simulink model "R7014E_DoubleTankSim"  (R2024b)
settings: Solver=ode5  StartTime=0.0  StopTime=2000  FixedStep=Ts  RelTol=1e-3  EnableMultiTasking=on
undefined symbols (not defined in the file): Ad, Bd, Cd, h_10, h_20, K, Q, T, Ts, u0
libraries: simulink x3, cstblocks x1
Description:
  | Double tank process simulation model
  | V1.0
  | 
  | Author: Wolfgang Birk, LTU
settings Model: MinMaxOverflowLogging=ForceOff  Creator=wolfgang  LastModifiedBy=Amar
settings SolverCC: AlgebraicLoopSolver=TrustRegion
settings DataIOCC: LimitDataPoints=on  SaveFormat=Array  SignalLoggingSaveFormat=ModelDataLogs  ReturnWorkspaceOutputs=off
settings OptimizationCC: ExpressionDepthLimit=2147483647  LifeSpan=inf
settings DebuggingCC: UnderspecifiedInitializationDetection=Classic  MergeDetectMultiDrivingBlocksExec=none  SolverPrmCheckMsg=warning  FcnCallInpInsideContextMsg=warning  UnconnectedInputMsg=warning  UnconnectedOutputMsg=warning  UnconnectedLineMsg=warning  StateNameClashWarn=warning  SFUnexpectedBacktrackingDiag=warning  SFNoUnconditionalDefaultTransitionDiag=warning  SFExecutionAtInitializationDiag=none  ArithmeticOperatorsInVariantConditions=warning
settings HardwareCC: ProdBitPerPointer=32  ProdBitPerSizeT=32  ProdBitPerPtrDiffT=32  ProdLargestAtomicFloat=None  ProdIntDivRoundTo=Undefined  ProdEndianess=Unspecified  ProdWordSize=32  ProdHWDeviceType=32-bit Generic
settings ModelReferenceCC: EnableRefExpFcnMdlSchedulingChecks=on  PropagateSignalLabelsOutOfModel=off
settings SFSimCC: SimUseLocalCustomCode=off  CustomCodeUndefinedFunction=UseInterfaceOnly
settings RTWCC: RTWUseLocalCustomCode=off  GPUComputeCapability=3.5
settings CodeAppCC: StateflowObjectComments=on
settings GRTTargetCC: TargetLangStandard=C89/C90 (ANSI)
settings ConfigComp: CovMetricSettings=dw  CovSaveCumulativeToWorkspaceVar=on  CovSaveSingleToWorkspaceVar=on  CovExternalEMLEnable=off

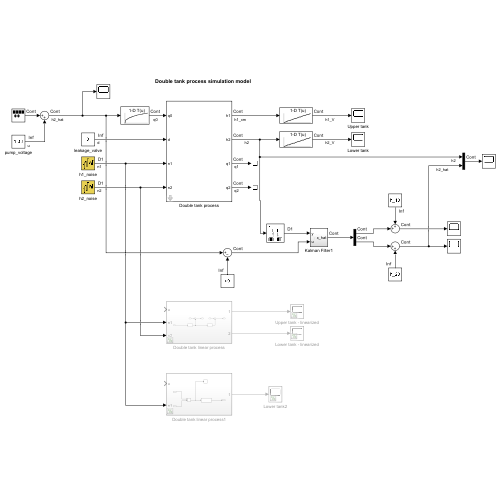
[thumbnail: Simulink's stored preview of the top-level diagram]
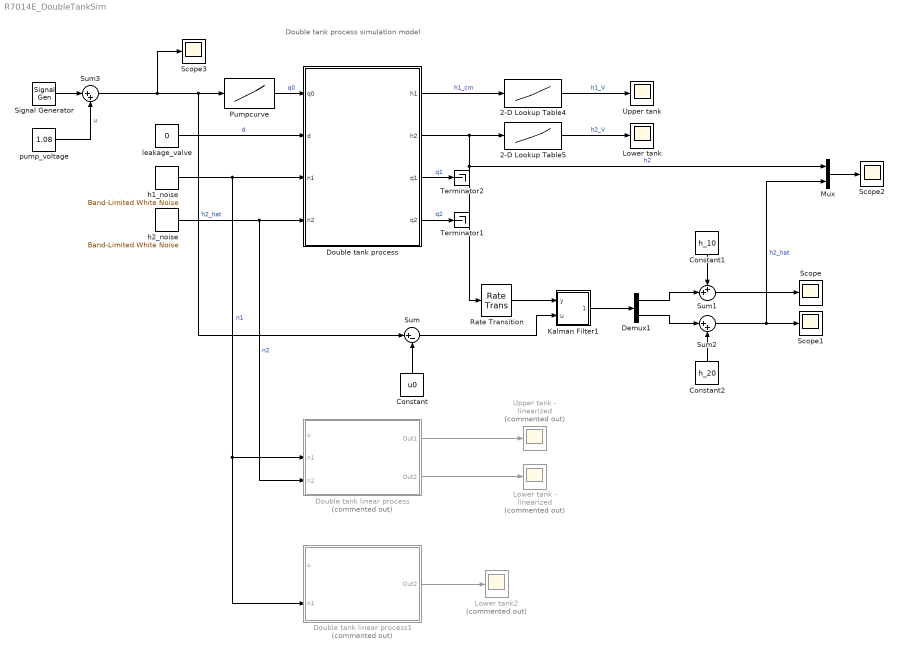
== system R7014E_DoubleTankSim ==
  note: Double tank process simulation model
  2-D Lookup Table4 : Lookup_n-D  NumberOfTableDimensions=1  BreakpointsForDimension1=x  BreakpointsForDimension2=[1:3]  Table=y  RndMeth=Simplest  mask{x=[2.50,3.00,3.50,4.00,4.50,5.00,5.50,6.00,6.50,7.00,7.50,8.00,8.50,9.00,9.50,10.00,10.50,11.00,11.50,12.00,12.50,13.00,13.50,14.00,14.50,15.00,15.50], y=[0.21,0.62,1.00,1.49,1.80,2.12,2.54,2.97,3.32,3.71,4.09,4.51,4.87,5.25,5.57,6.04,6.41,6.78,7.13,7.56,7.91,8.32,8.69,9.07,9.42,9.82,9.99]}
      mask prompts: x "Values on x-axis"; y "Values on y-axis"
  2-D Lookup Table5 : Lookup_n-D  NumberOfTableDimensions=1  BreakpointsForDimension1=x  BreakpointsForDimension2=[1:3]  Table=y  RndMeth=Simplest  mask{x=[2.50,3.00,3.50,4.00,4.50,5.00,5.50,6.00,6.50,7.00,7.50,8.00,8.50,9.00,9.50,10.00,10.50,11.00,11.50,12.00,12.50,13.00,13.50,14.00,14.50,15.00,15.50], y=[0.10,0.47,0.87,1.23,1.57,1.98,2.41,2.77,3.16,3.53,3.94,4.32,4.71,5.10,5.46, 5.85, 6.24, 6.63, 7.02, 7.42, 7.74, 8.15, 8.52, 8.90, 9.28, 9.67, 9.94]}
      mask prompts: x "Values on x-axis"; y "Values on y-axis"
  Constant : Constant  Value=u0
  Constant1 : Constant  Value=h_10
  Constant2 : Constant  Value=h_20
  Demux1 : Demux  Outputs=2
  Double tank linear process : Subsystem  Commented=on
  Double tank linear process1 : Subsystem  Commented=on
  Double tank process : Subsystem  mask{At=33, Ao=0.17, hmax=15.5}
      mask prompts: At "Tank area (cm^2)"; Ao "Opening area (cm^2)"; hmax "Tank height (cm)"
      mask help: Double tank process parameters
  Kalman Filter1 : Subsystem
  Lower tank : Scope
  Lower tank - linearized : Scope  Commented=on
  Lower tank2 : Scope  Commented=on
  Mux : Mux  Inputs=2
  Pumpcurve : Lookup_n-D  NumberOfTableDimensions=1  BreakpointsForDimension1=x  BreakpointsForDimension2=[1:3]  Table=y  RndMeth=Simplest  mask{x=[0,0.5,1,1.5,2,2.5,3,3.5,5,8,10], y=[0,16.47,20.75,24.52,27.63,30.06,32.49,34.80,40.28,48.24,52.43]}
      mask prompts: x "Values on x-axis"; y "Values on y-axis"
  Rate Transition : RateTransition  OutPortSampleTimeOpt=Inherit
  Scope{,1..3} (4 alike) : Scope
  Signal Generator : SignalGenerator  WaveForm=square  Amplitude=0.1  Frequency=0.001
  Sum : Sum  Inputs=|+-
  Sum1 : Sum  Inputs=++|
  Sum2 : Sum  Inputs=|++
  Sum3 : Sum  Inputs=|++
  Terminator1 : Terminator
  Terminator2 : Terminator
  Upper tank : Scope
  Upper tank - linearized : Scope  Commented=on
  h1_noise : simulink/Sources/Band-Limited White Noise  Cov=[2e-6]  Ts=Ts  seed=[23341]
  h2_noise : simulink/Sources/Band-Limited White Noise  Cov=[2e-6]  Ts=Ts  seed=[23341]
  leakage_valve : Constant  Value=0
  pump_voltage : Constant  Value=1.08
  wires:
  2-D Lookup Table4/1 -> Upper tank/1  "h1_V"
  leakage_valve/1 -> Double tank process/2(d)  "d"
  pump_voltage/1 -> Sum3/2  "u"
  Pumpcurve/1 -> Double tank process/1(q0)  "q0"
  Double tank process/1(h1) -> 2-D Lookup Table4/1  "h1_cm"
  Double tank process/2(h2) -> Rate Transition/1, Mux/1, 2-D Lookup Table5/1  "h2"
  Double tank process/4(q2) -> Terminator1/1  "q2"
  2-D Lookup Table5/1 -> Lower tank/1  "h2_V"
  Double tank process/3(q1) -> Terminator2/1  "q1"
  h1_noise/1 -> Double tank linear process1/2(n1), Double tank linear process/2(n1), Double tank process/3(n1)  "n1"
  h2_noise/1 -> Double tank linear process/3(n2), Double tank process/4(n2)  "n2"
  Double tank linear process/1(Out1) -> Upper tank - linearized/1
  Double tank linear process/2(Out2) -> Lower tank - linearized/1
  Double tank linear process1/1(Out2) -> Lower tank2/1
  Rate Transition/1 -> Kalman Filter1/1(y)
  Constant/1 -> Sum/2
  Sum/1 -> Kalman Filter1/2(u)
  Kalman Filter1/1(x_hat) -> Demux1/1
  Demux1/1 -> Sum1/2
  Constant1/1 -> Sum1/1
  Sum1/1 -> Scope/1
  Demux1/2 -> Sum2/1
  Constant2/1 -> Sum2/2
  Sum2/1 -> Mux/2, Scope1/1  "h2_hat"
  Mux/1 -> Scope2/1
  Sum3/1 -> Scope3/1, Sum/1, Pumpcurve/1  "h2_hat"
  Signal Generator/1 -> Sum3/1

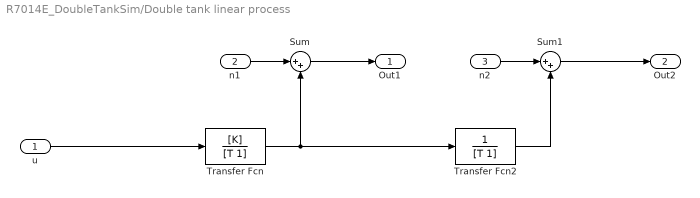
== system R7014E_DoubleTankSim/Double tank linear process ==
  u : Inport
  n1 : Inport  Port=2
  n2 : Inport  Port=3
  Sum : Sum  Inputs=|++
  Sum1 : Sum  Inputs=|++
  Transfer Fcn : TransferFcn  Numerator=[K]  Denominator=[T 1]
  Transfer Fcn2 : TransferFcn  Denominator=[T 1]
  Out1 : Outport
  Out2 : Outport  Port=2
  wires:
  n2/1 -> Sum1/1
  Sum/1 -> Out1/1
  Transfer Fcn/1 -> Transfer Fcn2/1, Sum/2
  Sum1/1 -> Out2/1
  n1/1 -> Sum/1
  u/1 -> Transfer Fcn/1
  Transfer Fcn2/1 -> Sum1/2

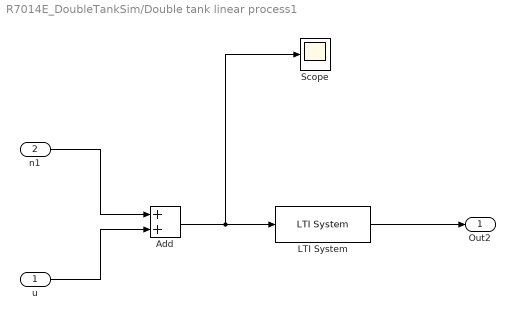
== system R7014E_DoubleTankSim/Double tank linear process1 ==
  u : Inport
  n1 : Inport  Port=2
  Add : Sum
  LTI System : cstblocks/LTI System  sys=sys  IC=[]  PadeOrder=0
  Scope : Scope
  Out2 : Outport
  wires:
  n1/1 -> Add/1
  LTI System/1 -> Out2/1
  u/1 -> Add/2
  Add/1 -> Scope/1, LTI System/1

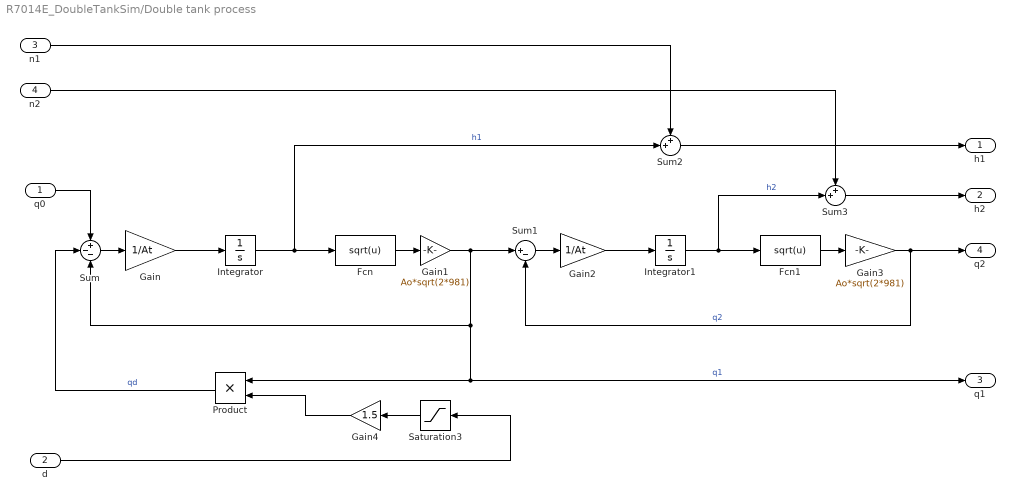
== system R7014E_DoubleTankSim/Double tank process ==
  q0 : Inport
  d : Inport  Port=2
  n1 : Inport  Port=3
  n2 : Inport  Port=4
  Fcn : Fcn  Expr=sqrt(u)
  Fcn1 : Fcn  Expr=sqrt(u)
  Gain : Gain  Gain=1/At
  Gain1 : Gain  Gain=Ao*sqrt(2*981)
  Gain2 : Gain  Gain=1/At
  Gain3 : Gain  Gain=Ao*sqrt(2*981)
  Gain4 : Gain  Gain=1.5
  Integrator : Integrator  LimitOutput=on  UpperSaturationLimit=hmax  LowerSaturationLimit=0
  Integrator1 : Integrator  LimitOutput=on  UpperSaturationLimit=hmax  LowerSaturationLimit=0
  Product : Product  RndMeth=Zero
  Saturation3 : Saturate  UpperLimit=1  LowerLimit=0
  Sum : Sum  Inputs=+--
  Sum1 : Sum  Inputs=|+-
  Sum2 : Sum  Inputs=++|
  Sum3 : Sum  Inputs=++|
  h1 : Outport  VectorParamsAs1DForOutWhenUnconnected=off
  h2 : Outport  Port=2  VectorParamsAs1DForOutWhenUnconnected=off
  q1 : Outport  Port=3  VectorParamsAs1DForOutWhenUnconnected=off
  q2 : Outport  Port=4  VectorParamsAs1DForOutWhenUnconnected=off
  wires:
  Sum/1 -> Gain/1
  Gain/1 -> Integrator/1
  Fcn/1 -> Gain1/1
  Gain1/1 -> Sum1/1, Product/1, q1/1, Sum/3  "q1"
  Sum1/1 -> Gain2/1
  Gain2/1 -> Integrator1/1
  Fcn1/1 -> Gain3/1
  Gain3/1 -> Sum1/2, q2/1  "q2"
  q0/1 -> Sum/1
  Integrator/1 -> Sum2/2, Fcn/1  "h1"
  Product/1 -> Sum/2  "qd"
  d/1 -> Saturation3/1
  Integrator1/1 -> Sum3/2, Fcn1/1  "h2"
  Saturation3/1 -> Gain4/1
  Gain4/1 -> Product/2
  Sum2/1 -> h1/1
  n1/1 -> Sum2/1
  Sum3/1 -> h2/1
  n2/1 -> Sum3/1

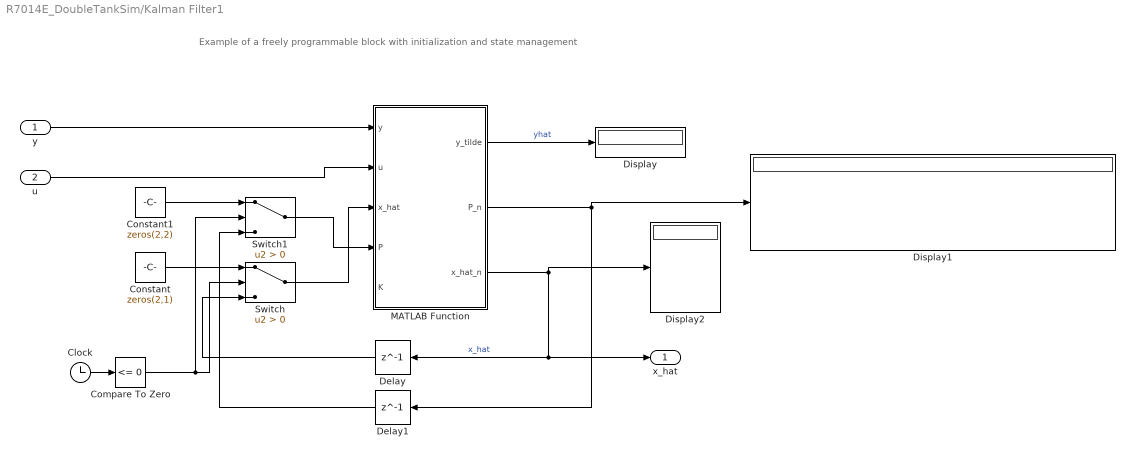
== system R7014E_DoubleTankSim/Kalman Filter1 ==
  note: Example of a freely programmable block with initialization and state management
  y : Inport
  u : Inport  Port=2
  Clock : Clock
  Compare To Zero : simulink/Logic and Bit Operations/Compare To Zero  relop=<=  OutDataTypeStr=boolean
  Constant : Constant  Value=zeros(2,1)
  Constant1 : Constant  Value=zeros(2,2)
  Delay : Delay  DelayLength=1  InitialCondition=0
  Delay1 : Delay  DelayLength=1  InitialCondition=0
  Display : Display
  Display1 : Display
  Display2 : Display
  MATLAB Function : MATLAB Function  TreatAsAtomicUnit=on
  Switch : Switch  Criteria=u2 > Threshold  SaturateOnIntegerOverflow=off  InputSameDT=off
  Switch1 : Switch  Criteria=u2 > Threshold  SaturateOnIntegerOverflow=off  InputSameDT=off
  x_hat : Outport  PortDimensions=2
  wires:
  Delay/1 -> Switch/3
  Switch/1 -> MATLAB Function/3(x_hat)
  Constant1/1 -> Switch1/1
  Compare To Zero/1 -> Switch1/2, Switch/2
  MATLAB Function/3(x_hat_n) -> Display2/1, x_hat/1, Delay/1  "x_hat"
  Constant/1 -> Switch/1
  MATLAB Function/1(y_tilde) -> Display/1  "yhat"
  MATLAB Function/2(P_n) -> Display1/1, Delay1/1
  Clock/1 -> Compare To Zero/1
  Switch1/1 -> MATLAB Function/4(P)
  y/1 -> MATLAB Function/1(y)
  Delay1/1 -> Switch1/3
  u/1 -> MATLAB Function/2(u)

== matlab function R7014E_DoubleTankSim/Kalman Filter1/MATLAB Function ==
  data: y input; u input; x_hat input; y_tilde output; P input; P_n output; x_hat_n output; Ad parameter; Bd parameter; Cd parameter; K input; Q parameter
function [y_tilde, P_n, x_hat_n] = fcn(y, u, x_hat, P, Ad, Bd, Cd, K, Q)

% Predict
x_hat_n = Ad*x_hat + Bd*u;
P_n = Ad*P*Ad' + Q;

% Update
y_tilde = y - Cd*x_hat;
x_hat_n = x_hat_n + K*y_tilde;
P_n = (eye(2) - K*Cd)*P_n;
y_tilde = y - Cd*x_hat_n;
